simulink model "prob5_214869"  (R2020a)
settings: Solver=VariableStepAuto  StartTime=0.0  StopTime=10.0  RelTol=1e-3
PostLoadFcn:
  | R=10;
  | C=10;
model workspace (MAT data in the model file):
  C = 10
  R = 10
settings Model: Creator=sonal  LastModifiedBy=sonal

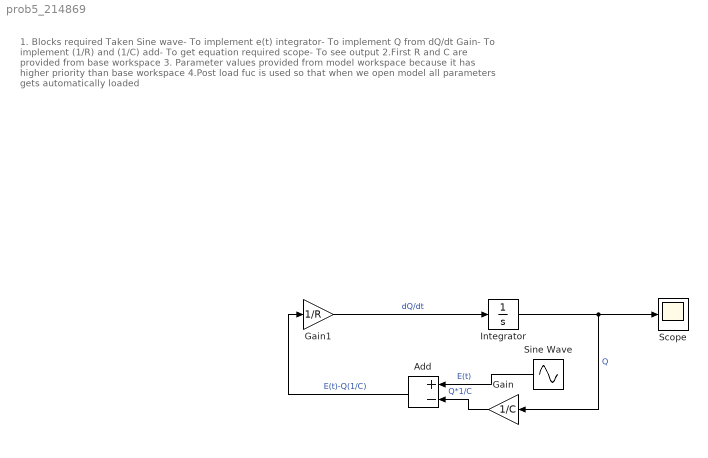
== system prob5_214869 ==
  note: 1. Blocks required Taken
      | Sine wave- To implement e(t)
      | integrator- To implement Q from dQ/dt
      | Gain- To implement (1/R) and (1/C)
      | add- To get equation required
      | scope- To see output
      |
      | 2.First R and C are provided from base workspace
      |
      | 3. Parameter values provided from model workspace because it has higher priority than base workspace
      |
      | 4.Post load fuc is used so that when we open model all parameters gets automatically loaded
  Add : Sum  Inputs=+-
  Gain : Gain  Gain=1/C
  Gain1 : Gain  Gain=1/R
  Integrator : Integrator  InitialCondition=10
  Scope : Scope
  Sine Wave : Sin  Amplitude=20  SampleTime=0
  wires:
  Sine Wave/1 -> Add/1  "E(t)"
  Gain/1 -> Add/2  "Q*1/C"
  Integrator/1 -> Gain/1, Scope/1  "Q"
  Add/1 -> Gain1/1  "E(t)-Q(1/C)"
  Gain1/1 -> Integrator/1  "dQ/dt"
